simulink model "ode_solver_2d"  (R2023a)
settings: Solver=VariableStepAuto  StartTime=0.0  StopTime=10.0  RelTol=1e-3
settings Model: Creator=joaog  LastModifiedBy=joaog

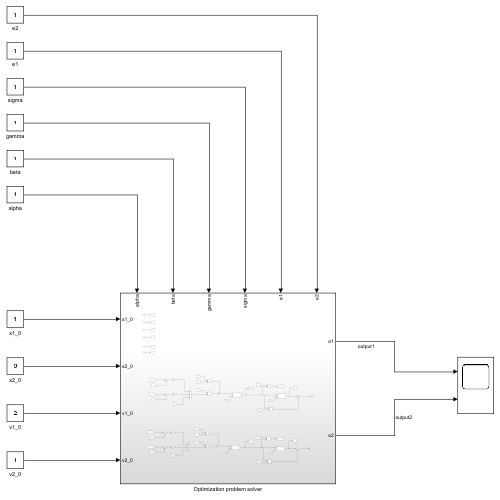
[thumbnail: Simulink's stored preview of the top-level diagram]
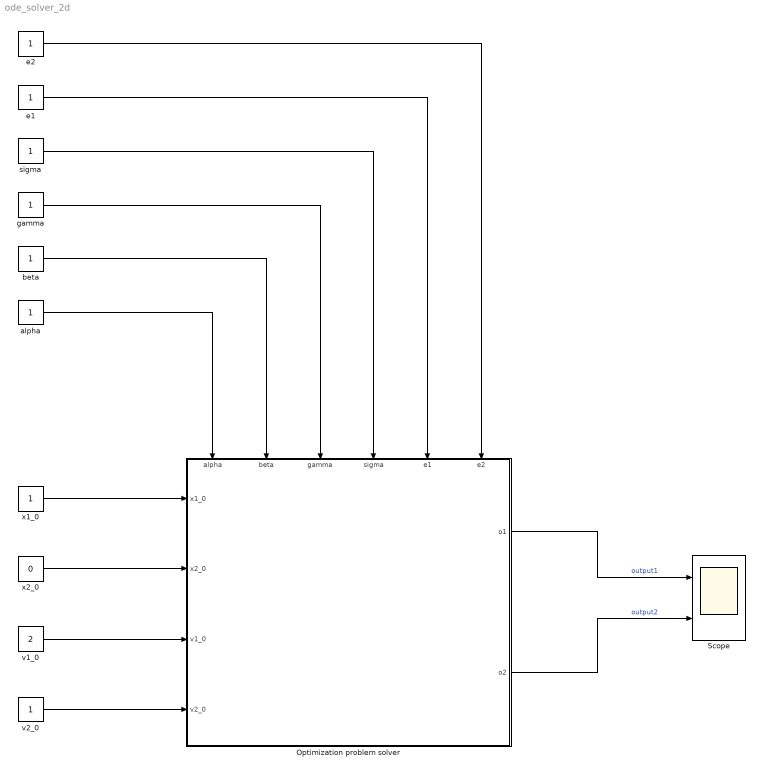
== system ode_solver_2d ==
  Optimization problem solver : Subsystem
      settings: PortSchema="{\"entries\":[{\"content\":{\"sides\":[{\"content\":{\"connectorIds\":[\"In1\",\"In2\",\"In3\",\"In4\"]},\"type\":\"ConnectorPlacement.EquallySpacedRectSide\",\"uuid\":\"ace58a2b-4bbe-49a2-915d-fce3e7b8fef9\"},{\"content\":{\"connectorIds\":[\"Out1\",\"Out2\"],\"side\":\"RIGHT\"},\"type\":\"ConnectorPlacement.EquallySpacedRectSide\",\"uuid\":\"d7f2c16b-5f0e-4f62-a2af-5253be17176a\"},{\"content\":{\"connectorIds\":[\"In5\",\"In6\",\"In7\",\"In8\",\"In9\",\"In10\"],\"side\":\"TOP\"},\"type\":\"ConnectorPlacement.EquallySpacedRectSide\",\"uuid\":\"f696cb1b-8c75-4876-acf7-079715f4e536\"}]},\"type\":\"ConnectorPlacement.EquallySpacedConnector\",\"uuid\":\"3d890d1a-9284-4c35-bb22-db42113889f5\"}],\"packageUris\":[\"http://schema.mathworks.com/mf0/Connector/R2020b\"],\"version\":\"1.0\"}"
  Scope : Scope  NumInputPorts=2
  alpha : Constant
  beta : Constant
  e1 : Constant
  e2 : Constant
  gamma : Constant
  sigma : Constant
  v1_0 : Constant  Value=2
  v2_0 : Constant
  x1_0 : Constant
  x2_0 : Constant  Value=0
  wires:
  alpha/1 -> Optimization problem solver/5(alpha)
  beta/1 -> Optimization problem solver/6(beta)
  gamma/1 -> Optimization problem solver/7(gamma)
  sigma/1 -> Optimization problem solver/8(sigma)
  e1/1 -> Optimization problem solver/9(e1)
  e2/1 -> Optimization problem solver/10(e2)
  x1_0/1 -> Optimization problem solver/1(x1_0)
  x2_0/1 -> Optimization problem solver/2(x2_0)
  v1_0/1 -> Optimization problem solver/3(v1_0)
  v2_0/1 -> Optimization problem solver/4(v2_0)
  Optimization problem solver/1(o1) -> Scope/1  "output1"
  Optimization problem solver/2(o2) -> Scope/2  "output2"

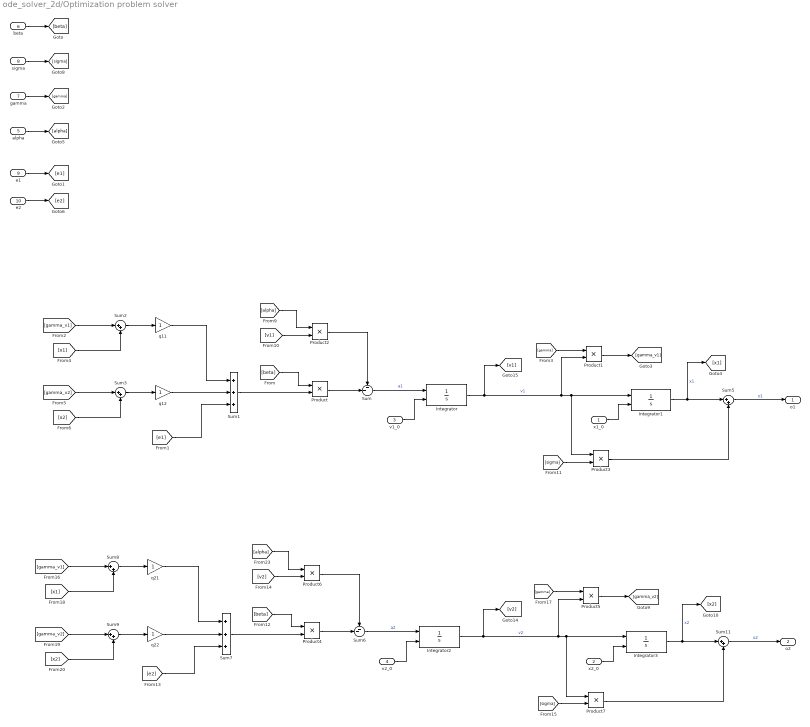
== system ode_solver_2d/Optimization problem solver ==
  x1_0 : Inport
  x2_0 : Inport  Port=2
  v1_0 : Inport  Port=3
  v2_0 : Inport  Port=4
  alpha : Inport  Port=5
  beta : Inport  Port=6
  gamma : Inport  Port=7
  sigma : Inport  Port=8
  e1 : Inport  Port=9
  e2 : Inport  Port=10
  Integrator{,1..3} (4 alike) : Integrator  InitialConditionSource=external
  Product{,1..7} (8 alike) : Product
  Sum : Sum  Inputs=--|
  Sum1 : Sum  Inputs=+++
  Sum{2..3,5,8..9,11} (6 alike) : Sum  Inputs=|++
  Sum6 : Sum  Inputs=--|
  Sum7 : Sum  Inputs=+++
  q{11..12,21..22} (4 alike) : Gain
  o1 : Outport
  o2 : Outport  Port=2
  wires:
  [gamma_v1] -> Sum8/1
  Sum8/1 -> q21/1
  Integrator/1 -> [v1], Integrator1/1, Product3/1, Product1/2  "v1"
  Product7/1 -> Sum11/2
  q12/1 -> Sum1/2
  Integrator3/1 -> [x2], Sum11/1  "x2"
  [gamma_v2] -> Sum9/1
  [beta] -> Product4/1
  Sum1/1 -> Product/2
  [beta] -> Product/1
  Sum7/1 -> Product4/2
  sigma/1 -> [sigma]
  Product/1 -> Sum/2
  Integrator2/1 -> [v2], Product5/2, Integrator3/1, Product7/1  "v2"
  [gamma_v1] -> Sum2/1
  Sum9/1 -> q22/1
  Sum5/1 -> o1/1  "o1"
  q21/1 -> Sum7/1
  beta/1 -> [beta]
  Product1/1 -> [gamma_v1]
  [x2] -> Sum9/2
  Sum3/1 -> q12/1
  e1/1 -> [e1]
  Product3/1 -> Sum5/2
  [alpha] -> Product6/1
  e2/1 -> [e2]
  Sum/1 -> Integrator/1  "a1"
  Integrator1/1 -> [x1], Sum5/1  "x1"
  Product5/1 -> [gamma_v2]
  Sum6/1 -> Integrator2/1  "a2"
  [alpha] -> Product2/1
  x1_0/1 -> Integrator1/2
  q11/1 -> Sum1/1
  [v2] -> Product6/2
  Product4/1 -> Sum6/2
  Product6/1 -> Sum6/1
  Sum11/1 -> o2/1  "o2"
  [x1] -> Sum2/2
  v2_0/1 -> Integrator2/2
  x2_0/1 -> Integrator3/2
  [x1] -> Sum8/2
  alpha/1 -> [alpha]
  [gamma_v2] -> Sum3/1
  [gamma] -> Product5/1
  [gamma] -> Product1/1
  [sigma] -> Product7/2
  q22/1 -> Sum7/2
  [x2] -> Sum3/2
  Sum2/1 -> q11/1
  gamma/1 -> [gamma]
  [sigma] -> Product3/2
  Product2/1 -> Sum/1
  [v1] -> Product2/2
  v1_0/1 -> Integrator/2
  [e2] -> Sum7/3
  [e1] -> Sum1/3
